simulink subsystem "FTs_Piero"  (R2024b)
settings: Solver=VariableStepAuto  StartTime=0.0  StopTime=10.0  RelTol=1e-3
settings Model: Creator=Chenfu  LastModifiedBy=Chenfu

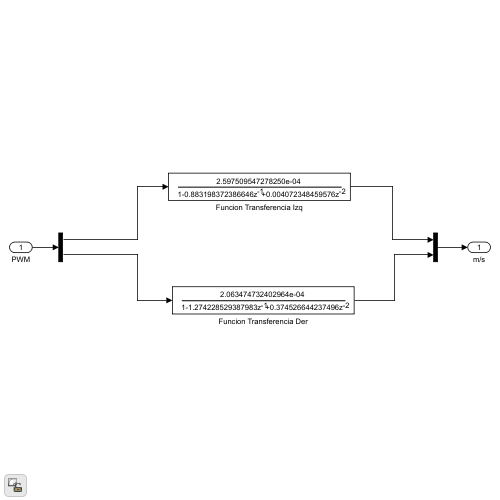
[thumbnail: Simulink's stored preview of the top-level diagram]
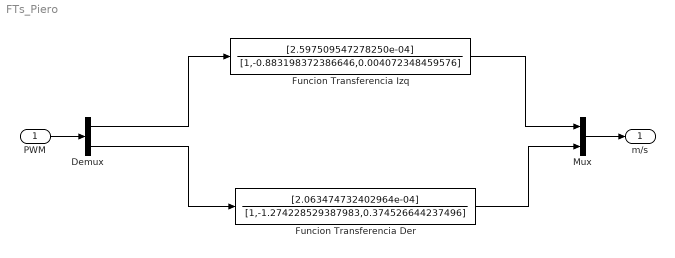
== system FTs_Piero ==
  PWM : Inport
  Demux : Demux  Outputs=2
  Funcion Transferencia Der : DiscreteFilter  Numerator=[2.063474732402964e-04]  Denominator=[1,-1.274228529387983,0.374526644237496]
  Funcion Transferencia Izq : DiscreteFilter  Numerator=[2.597509547278250e-04]  Denominator=[1,-0.883198372386646,0.004072348459576]
  Mux : Mux  Inputs=2
  m/s : Outport
  wires:
  PWM/1 -> Demux/1
  Mux/1 -> m/s/1
  Demux/1 -> Funcion Transferencia Izq/1
  Demux/2 -> Funcion Transferencia Der/1
  Funcion Transferencia Der/1 -> Mux/2
  Funcion Transferencia Izq/1 -> Mux/1
